simulink model "PUNTO"  (Simulink 9.0)
settings: Solver=VariableStepAuto  StartTime=0.0  StopTime=10.0  RelTol=1e-3
settings Model: Creator=ruiso  LastModifiedBy=ruiso
settings DataIOCC: SaveFormat=Dataset
settings OptimizationCC: LifeSpan=auto
settings DebuggingCC: UnderspecifiedInitializationDetection=Simplified  MergeDetectMultiDrivingBlocksExec=error  SFUnexpectedBacktrackingDiag=error  SFNoUnconditionalDefaultTransitionDiag=error  SFExecutionAtInitializationDiag=warning
settings HardwareCC: ProdBitPerPointer=64  ProdBitPerSizeT=64  ProdBitPerPtrDiffT=64  ProdLargestAtomicFloat=Float  ProdIntDivRoundTo=Zero  ProdEndianess=LittleEndian  ProdWordSize=64  ProdHWDeviceType=Intel->x86-64 (Windows64)
settings ModelReferenceCC: PropagateSignalLabelsOutOfModel=on
settings CodeAppCC: StateflowObjectComments=off
settings GRTTargetCC: TargetLangStandard=C99 (ISO)
settings ConfigComp: CovMetricSettings=dwe  CovHtmlReporting=off  CovSaveCumulativeToWorkspaceVar=off  CovSaveSingleToWorkspaceVar=off  CovExternalEMLEnable=on

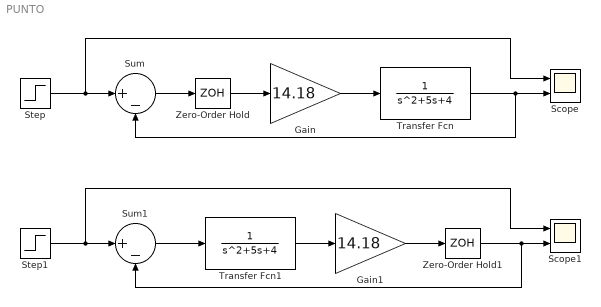
== system PUNTO ==
  Gain : Gain  Gain=14.18
  Gain1 : Gain  Gain=14.18
  Scope : Scope  NumInputPorts=2
  Scope1 : Scope  NumInputPorts=2
  Step : Step  SampleTime=0
  Step1 : Step  SampleTime=0
  Sum : Sum  Inputs=|+-
  Sum1 : Sum  Inputs=|+-
  Transfer Fcn : TransferFcn  Denominator=[1 5 4]
  Transfer Fcn1 : TransferFcn  Denominator=[1 5 4]
  Zero-Order Hold : ZeroOrderHold  SampleTime=-1
  Zero-Order Hold1 : ZeroOrderHold  SampleTime=-1
  wires:
  Transfer Fcn/1 -> Sum/2, Scope/2
  Gain/1 -> Transfer Fcn/1
  Zero-Order Hold/1 -> Gain/1
  Sum/1 -> Zero-Order Hold/1
  Step/1 -> Sum/1, Scope/1
  Step1/1 -> Sum1/1, Scope1/1
  Transfer Fcn1/1 -> Gain1/1
  Sum1/1 -> Transfer Fcn1/1
  Gain1/1 -> Zero-Order Hold1/1
  Zero-Order Hold1/1 -> Sum1/2, Scope1/2
